simulink model "adcD"  (R2022b)
settings: Solver=VariableStepAuto  StartTime=0.0  StopTime=1  RelTol=1e-3
libraries: dspstat3 x6, instrumentseriallib x2
settings Model: SimulationMode=accelerator  Creator=ASUS  LastModifiedBy=ASUS

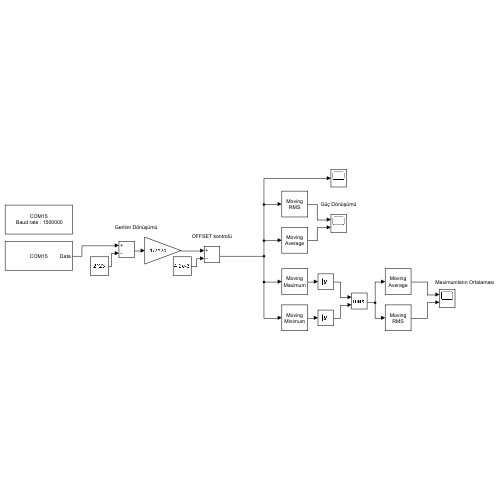
[thumbnail: Simulink's stored preview of the top-level diagram]
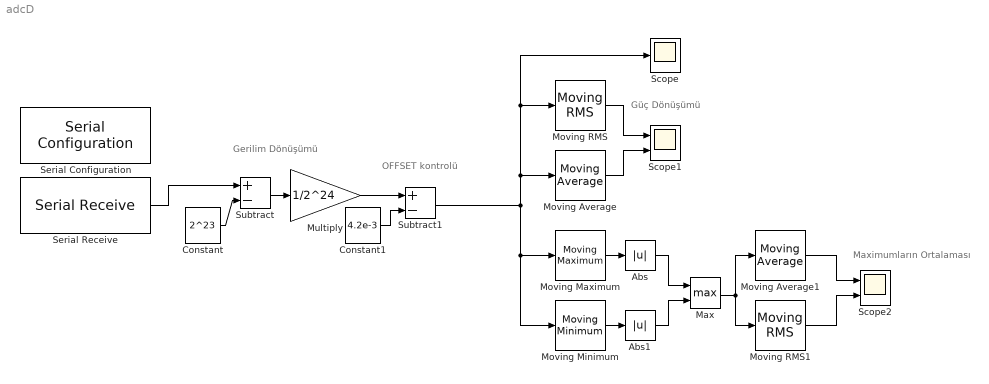
== system adcD ==
  note: OFFSET kontrolü
  note: Gerilim Dönüşümü
  note: Güç Dönüşümü
  note: Maximumların Ortalaması
  Abs : Abs  SaturateOnIntegerOverflow=off
  Abs1 : Abs  SaturateOnIntegerOverflow=off
  Constant : Constant  Value=2^23
  Constant1 : Constant  Value=4.2e-3
  Max : MinMax  Function=max  Inputs=2
  Moving Average : dspstat3/Moving Average  Method=Sliding window  ForgettingFactorPort=off  SpecifyWindowLength=on  WindowLength=60  OverlapLength=59  AllowArbitraryInputLength=on  ForgettingFactor=0.9  SimulateUsing=Code generation
  Moving Average1 : dspstat3/Moving Average  Method=Sliding window  ForgettingFactorPort=off  SpecifyWindowLength=on  WindowLength=4  OverlapLength=3  AllowArbitraryInputLength=on  ForgettingFactor=0.9  SimulateUsing=Code generation
  Moving Maximum : dspstat3/Moving Maximum  SpecifyWindowLength=on  WindowLength=240  SimulateUsing=Code generation
  Moving Minimum : dspstat3/Moving Minimum  SpecifyWindowLength=on  WindowLength=240  SimulateUsing=Code generation
  Moving RMS : dspstat3/Moving RMS  Method=Sliding window  ForgettingFactorPort=off  SpecifyWindowLength=on  WindowLength=60  OverlapLength=59  AllowArbitraryInputLength=on  ForgettingFactor=0.9  SimulateUsing=Interpreted execution
  Moving RMS1 : dspstat3/Moving RMS  Method=Sliding window  ForgettingFactorPort=off  SpecifyWindowLength=on  WindowLength=4  OverlapLength=3  AllowArbitraryInputLength=on  ForgettingFactor=0.9  SimulateUsing=Interpreted execution
  Multiply : Gain  Gain=1/2^24
  Scope : Scope
  Scope1 : Scope  NumInputPorts=2
  Scope2 : Scope  NumInputPorts=2
  Serial Configuration : instrumentseriallib/Serial Configuration  Priority=-200000  PortSel=COM15  Port=COM15  ComPort=COM15  BaudRate=1500000  DataBits=8  Parity=none  StopBits=1  ByteOrder=little-endian  FlowControl=none  Timeout=1000000  SimulateUsing=Interpreted execution  BlockInModel=on  aMode=1
  Serial Receive : instrumentseriallib/Serial Receive  Priority=1  PortSel=COM15  Port=COM15  ComPort=COM15  DataType=uint32  SaveDataType=uint8  ToggleHeader=off  Header=[]  ToggleTerminator=on  Terminator=Custom terminator  CustomTerminator=[0xA5]  InputFormat=Column major  ToggleDataSize=on  DataSize=[1 1]  EnableBlockingMode=on  ActionDataUnavailable=Output last received value  ActionWhenDataUnavailable=Output last received value  CustomValue=0  SampleTime=1/(30000)  SimulateUsing=Interpreted execution  BlockInModel=on  aMode=1
  Subtract : Sum  Inputs=+-
  Subtract1 : Sum  Inputs=+-
  wires:
  Constant/1 -> Subtract/2
  Subtract/1 -> Multiply/1
  Serial Receive/1 -> Subtract/1
  Moving RMS/1 -> Scope1/1
  Multiply/1 -> Subtract1/1
  Constant1/1 -> Subtract1/2
  Subtract1/1 -> Moving RMS/1, Scope/1, Moving Average/1, Moving Minimum/1, Moving Maximum/1
  Moving Maximum/1 -> Abs/1
  Moving Minimum/1 -> Abs1/1
  Abs/1 -> Max/1
  Abs1/1 -> Max/2
  Max/1 -> Moving RMS1/1, Moving Average1/1
  Moving Average/1 -> Scope1/2
  Moving Average1/1 -> Scope2/1
  Moving RMS1/1 -> Scope2/2
